simulink model "TireSoilInteractionTestHarness"  (R2024a)
settings: Solver=VariableStepAuto  StartTime=0.0  StopTime=100  RelTol=1e-3
libraries: fl_lib x12, nesl_utility x2, sdl_lib x1
settings Model: Creator=asakhare  LastModifiedBy=asakhare
settings SimscapeCC: SimscapeLogType=all

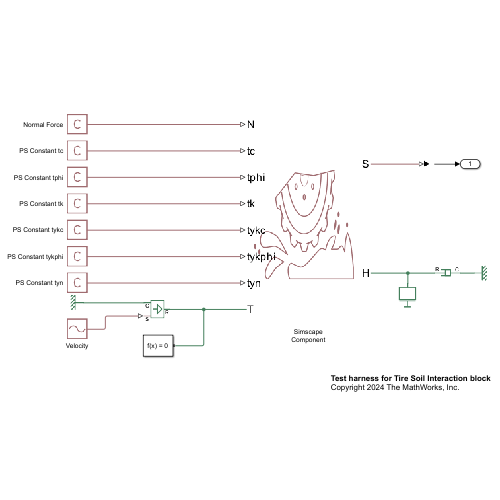
[thumbnail: Simulink's stored preview of the top-level diagram]
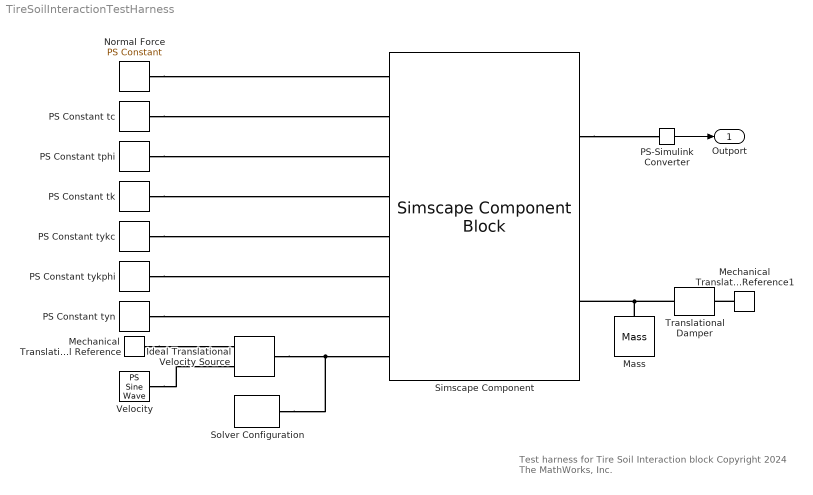
== system TireSoilInteractionTestHarness ==
  note: Test harness for Tire Soil Interaction block
      | Copyright 2024 The MathWorks, Inc.
  Ideal Translational Velocity Source : fl_lib/Mechanical/Mechanical Sources/Ideal Translational Velocity Source
  Mass : fl_lib/Mechanical/Translational Elements/Mass  mass=10 kg  num_ports=foundation.enum.numPorts2.one  v_specify=off  v_priority=High  v=.5 m/s  v_nominal_specify=off  v_nominal_value=1  v_nominal_unit=m/s  f_specify=off  f_priority=None  f=0 N  f_nominal_specify=off  f_nominal_value=1  f_nominal_unit=N
  Mechanical Translational Reference : fl_lib/Mechanical/Translational Elements/Mechanical Translational Reference
  Mechanical Translational Reference1 : fl_lib/Mechanical/Translational Elements/Mechanical Translational Reference
  Normal Force : fl_lib/Physical Signals/Sources/PS Constant  constant=100 N
  PS Constant tc : fl_lib/Physical Signals/Sources/PS Constant  constant=1000 N/m^2
  PS Constant tk : fl_lib/Physical Signals/Sources/PS Constant  constant=0.1 m
  PS Constant tphi : fl_lib/Physical Signals/Sources/PS Constant  constant=60 deg
  PS Constant tykc : fl_lib/Physical Signals/Sources/PS Constant  constant=48
  PS Constant tykphi : fl_lib/Physical Signals/Sources/PS Constant  constant=6076
  PS Constant tyn : fl_lib/Physical Signals/Sources/PS Constant  constant=0.78
  PS-Simulink Converter : nesl_utility/PS-Simulink Converter  PhysicalDomain=network_engine_domain  SubClassName=ps_output  LeftPortType=input  RightPortType=output  PseudoPeriodic=off  Frequencies=[]  VectorFormat=inherit  Unit=inherit  AffineConversion=off
  Simscape Component : SimscapeComponentBlock  SourceFile=tire_soil_interaction  ComponentPath=tire_soil_interaction  ComponentVariants="[\"tire_soil_interaction\"]"  ComponentVariantNames="[\"tire_soil_interaction\"]"  ClassName=tire_soil_interaction  SchemaVersion=1  load_TLU=[2.225, 4.45, 6.6725, 8.9, 11.125, 13.35] kN  p_inflation_TLU=[69, 138, 207, 276, 345] kPa  deflection_TLU=[1.896, 1.239, 1.021, .894, .776; 3.623, 2.423, 1.963, 1.64, 1.435; 5.119, 3.477, 2.77, 2.311, 2.008; 6.447, 4.413, 3.528, 2.939, 2.533; 7.917, 5.306, 4.191, 2.494, 3.03; 9.169, 6.098, 4.851, 4.059, 3.494] cm  area_TLU=[179.93, 145.82, 127.81, 102.68, 100.92; 517.26, 262.89, 211.79, 182.92, 165.86; 726.09, 424.44, 304.42, 241.47, 233.76; 947.36, 604.21, 414.85, 343.35, 297.14; 1085.95, 749.58, 556.91, 443.03, 372.77; 1214.12, 865.65, 649.45, 525.61, 445.5] cm^2  inflation_pressure=100 kPa  r_e_t=0.5 m  bti=0.327 m  hti=0.245 m  k_e=7  vxlow=1 m/s  v_tr_thr=0.001 m/s  kpumin=-1  kpumax=1  p_thr=0.01 bar  b_thr=1 mm
      settings: CopyFcn=simscape.engine.sli.internal.componentblockcallback(gcbh,'COPY')  PreCopyFcn=simscape.engine.sli.internal.componentblockcallback(gcbh,'PRECOPY')  PreDeleteFcn=simscape.engine.sli.internal.componentblockcallback(gcbh,'PREDELETE')  InternalSimscapePortConfiguration="{\"Bottom\":[],\"Left\":[{\"id\":\"N\",\"label\":\"N\",\"type\":\"input\"},{\"id\":\"tc\",\"label\":\"tc\",\"type\":\"input\"},{\"id\":\"tphi\",\"label\":\"tphi\",\"type\":\"input\"},{\"id\":\"tk\",\"label\":\"tk\",\"type\":\"input\"},{\"id\":\"tykc\",\"label\":\"tykc\",\"type\":\"input\"},{\"id\":\"tykphi\",\"label\":\"tykphi\",\"type\":\"input\"},{\"id\":\"tyn\",\"label\":\"tyn\",\"type\":\"input\"},{\"id\":\"T\",\"label\":\"T\",\"type\":\"foundation.mechanical.translational.translational\"}],\"Right\":[{\"id\":\"S\",\"label\":\"S\",\"type\":\"output\"},{\"id\":\"H\",\"label\":\"H\",\"type\":\"foundation.mechanical.translational.translational\"}],\"Top\":[]}"
      mask Type: Tire-Soil Interaction (Based on Bekker equation implementation)
  Solver Configuration : nesl_utility/Solver Configuration  PhysicalDomain=network_engine_domain  SubClassName=solver  LeftPortType=input  RightPortType=generic  Tones=[]  Harmonics=[]  SimulateNoise=off  Profile=off  UseLocalSampling=off  EnableSwitchedLinearOptims=on  FrequencyDomain=off  UseCCode=off  RelTol=0.001  AbsTol=0.001  MinStep=1e-09  ToWorkspace=off  RevertToSquareIcSolve=off  NumHomotopyIterations=100  PhasorMode=off  PhasorModeNumHarmonics=1  ConsistencySolver=NEWTON_XTOL_AFTER_FTOL  IndexReductionMethod=DerivativeReplacement  DoDC=off  ResidualTolerance=1e-09  ConsistencyTolSource=GLOBAL  ConsistencyAbsTol=0.001  ConsistencyRelTol=0.001  ConsistencyTolFactor=0.001  UseLocalSolver=off  LocalSolverChoice=NE_BACKWARD_EULER_ADVANCER  ResolveIndetEquations=on  FunctionEvalNumThread=1  LocalSolverSampleTime=0.001  DoFixedCost=off  MaxNonlinIter=3  MaxModeIter=2  ComputeImpulses=off  ImpulseIterations=2  LinearAlgebra=auto  LinearAlgebraNumThread=0  EquationFormulation=NE_TIME_EF  DelaysMemoryBudget=1024  AutomaticFiltering=on  FilteringTimeConstant=0.001  PartitionStorageMethod=AS_NEEDED  PartitionMemoryBudget=1024  PartitionMethod=ROBUST  MultibodyUseLocalSolver=off  MultibodyLocalSolverChoice=ODE1  MultibodyLocalSolverSampleTime=0.001
  Translational Damper : sdl_lib/Couplings & Drives/Springs & Dampers/Translational Damper  D=1e-3 N*s/m  enable_faults=simscape.enum.onoff.off  b_fault=1e6 N*s/m  fault_trigger=simscape.fault.triggertype.external  acceleration_limit=100 m/s^2  shock_limit=1  thermal_port=simscape.enum.thermaleffects.omit  thermal_mass=50 kJ/K  temperature_specify=off  temperature_priority=High  temperature=300 K  temperature_nominal_specify=off  temperature_nominal_value=1  temperature_nominal_unit=K
  Velocity : fl_lib/Physical Signals/Sources/PS Sine Wave  amplitude=5 m/s  bias=0 m/s  frequency_spec=foundation.enum.frequencySpec.frequencySI  frequency_SI=1/50 Hz  frequency_angular=1 rad/s  phase=0 rad
      settings: InternalSimscapePortConfiguration="{\"Bottom\":[],\"Left\":[],\"Right\":[{\"id\":\"O\",\"label\":\"\",\"type\":\"output\"}],\"Top\":[]}"
  Outport : Outport
  wires:
  PS-Simulink Converter/1 -> Outport/1
  connections:
  PS Constant tykc/RConn1 -- Simscape Component/LConn5
  PS Constant tykphi/RConn1 -- Simscape Component/LConn6
  PS Constant tyn/RConn1 -- Simscape Component/LConn7
  PS Constant tk/RConn1 -- Simscape Component/LConn4
  PS Constant tc/RConn1 -- Simscape Component/LConn2
  PS Constant tphi/RConn1 -- Simscape Component/LConn3
  Normal Force/RConn1 -- Simscape Component/LConn1
  Ideal Translational Velocity Source/LConn1 -- Simscape Component/LConn8 -- Solver Configuration/RConn1
  Mechanical Translational Reference/LConn1 -- Ideal Translational Velocity Source/RConn2
  Translational Damper/LConn1 -- Mass/LConn1 -- Simscape Component/RConn2
  Mechanical Translational Reference1/LConn1 -- Translational Damper/RConn1
  Simscape Component/RConn1 -- PS-Simulink Converter/LConn1
  Velocity/RConn1 -- Ideal Translational Velocity Source/RConn1
